simulink library "speedgoatlib_IO71X"  (R2012b)
settings: Solver=ode45  StartTime=0.0  StopTime=10.0  RelTol=1e-3
undefined symbols (not defined in the file): macaddr
Description:
  | 7.14.0.739 (R2012a)
settings Model: xpc_rtwmakecfg_data=_xpciplib__xpcetherlib__xpcether8255xlib__xpcnblib__xpcetherGbElib_  Creator=dkuratli  LastModifiedBy=lab3

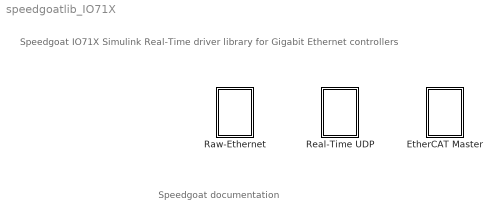
== system speedgoatlib_IO71X ==
  note: Speedgoat IO71X Simulink Real-Time driver library
      | for Gigabit Ethernet controllers
  note: Speedgoat documentation
  EtherCAT Master : Subsystem
      settings: OpenFcn=xpcethercatlib
  Raw-Ethernet : Subsystem
      settings: OpenFcn=xpcethernetlib
  Real-Time UDP : Subsystem

== system speedgoatlib_IO71X/EtherCAT Master ==

== system speedgoatlib_IO71X/Raw-Ethernet ==

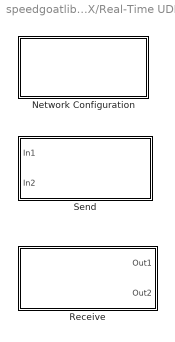
== system speedgoatlib_IO71X/Real-Time UDP ==
  "Network Configuration " : Subsystem  mask(xpcnwconfig){EthController=1, IpAddress=0.0.0.0, SubnetMask=255.255.255.0, Gateway=0.0.0.0, EthDrv=Intel Gigabit, PciBus=0, PciSlot=0, BufferSizes=[100 10 10 200]}
      mask prompts: EthController "Ethernet controller"; IpAddress "IP Address:"; SubnetMask "Subnet Mask:"; EthDrv "Ethernet Driver"; PciBus "PCI Bus:"; PciSlot "PCI Slot:"; BufferSizes "Buffer pool sizes (256, 512, 1024, 2048)"
      mask help: Network Configuration
      mask init:
      | EthDrv = 2;
      | IpAddress = ipaddr(IpAddress);
      | SubnetMask = ipaddr(SubnetMask);
      | Gateway = ipaddr(Gateway);
      mask Help: eval('xpcdoc(''RT_NETWORK_CONFIGURATION'')');
      mask TypeOptions EthController: 1 | 2 | 3 | 4 | 5 | 6 | 7 | 8 | 9 | 10
      mask TypeOptions EthDrv: Intel 8255x | Intel Gigabit
      mask Display: disp(['Speedgoat\nI8254x (IO71X)\nNetwork Configuration\nEthernet controller: ', num2str(EthController)]);
  "Receive " : Subsystem  mask(receive){EthController=1, Receive1=0.0.0.0, Receive2=25000, Receive3=1, Receive4=-1}
      mask prompts: EthController "Ethernet controller:"; Receive1 "IP address to receive from (0.0.0.0 for accepting all):"; Receive2 "IP port to receive from:"; Receive3 "Output port width:"; Receive4 "Sample time:"
      mask help: UDP Receive (adapted by Speedgoat)
      mask init:
      | Receive1 = ipaddr(Receive1);
      mask Help: helpview(fullfile(docroot, 'mapfiles', 'xpc.map'), 'RT_UDP_RECEIVE')
      mask TypeOptions EthController: 1 | 2 | 3 | 4 | 5 | 6 | 7 | 8 | 9 | 10
      mask Display: disp(['Speedgoat\nI8254x (IO71X)\nUDP Receive\nEthernet controller: ', num2str(EthController)])
  "Send " : Subsystem  mask(send){EthController=1, Send1=255.255.255.255, Send2=25000, Send3=-1, Send4=-1}
      mask prompts: EthController "Ethernet controller:"; Send1 "IP address to send to (255.255.255.255 for broadcast):"; Send2 "Remote IP port to send to:"; Send3 "Use the following local IP port (-1 for automatic assignment):"; Send4 "Sample time:"
      mask help: UDP Send (adapted by Speedgoat)
      mask init:
      | Send1 = ipaddr(Send1);
      mask Help: helpview(fullfile(docroot, 'mapfiles', 'xpc.map'), 'RT_UDP_SEND')
      mask TypeOptions EthController: 1 | 2 | 3 | 4 | 5 | 6 | 7 | 8 | 9 | 10
      mask Display: disp(['Speedgoat\nI8254x (IO71X)\nUDP Send\nEthernet controller: ',num2str(EthController)])

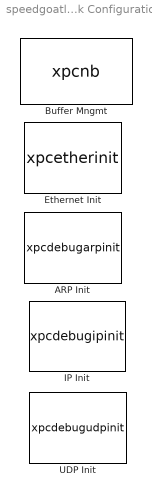
== system speedgoatlib_IO71X/Real-Time UDP/Network Configuration  ==
  "ARP Init " : S-Function  Priority=0  FunctionName=xpcdebugarpinit  Parameters=Stats, Interface, IpAddress, SubnetMask, Gateway, EthernetId, Flags, BlockId, Retry, Timeout, Expiration, StaticAddressListIp, StaticAddressListMac, DiscoveryList, MulticastList, SampleTime  EnableBusSupport=off  mask(arpinit){Interface=EthController-1, IpAddress=IpAddress, SubnetMask=SubnetMask, Gateway=Gateway, EthernetId=EthController, BlockId=EthController-1, SampleTime=-1, Flags=hex2dec('00000697'), Stats=off, Retry=5, Timeout=20, Expiration=20*60, StaticAddressListIp=[], StaticAddressListMac=[], DiscoveryList=[], MulticastList=[]}
      mask prompts: IpAddress "IP Address"; SubnetMask "Subnet Mask"; EthernetId "Ethernet ID"; BlockId "Block ID"; SampleTime "Sample Time"; Stats "Statistics Port"; StaticAddressListIp "[Static IP]"; StaticAddressListMac "[Static MAC]"; DiscoveryList "[Discovery IP]"; MulticastList "[Multicast IP]"
      mask help: ARP Init
      mask init:
      | xpclinklib('xpciplib');
      mask Help: web('arpdebug.htm',  '-helpbrowser');
      mask Display: disp('ARP Init');
  "Buffer Mngmt " : S-Function  Priority=-1  FunctionName=xpcnb  Parameters=pool_sizes, SampleTime, ShowTune  EnableBusSupport=off  mask(xpcnbinit){SampleTime=-1, PoolSizes=BufferSizes, ShowTune=on}
      mask prompts: SampleTime "Sample time:"; PoolSizes "Buffer pool sizes (256, 512, 1024, 2048):"; ShowTune "Display tuning information"
      mask help: Network Buffer Initialization
      mask init:
      | [MaskDisplay, pool_sizes] = mxpcnbinit(2, PoolSizes);
      | 
      | set_param(gcb, 'MaskDisplay', MaskDisplay);
      mask Help: eval('xpcdoc(''NB_Init'')');
      mask Display: disp('Network Buffer\nManagement');
  "Ethernet Init " : S-Function  Priority=-1  FunctionName=xpcetherinit  Parameters="ID, Driver, Bus, Slot, VendorID, DeviceID, AddressSource, mac, TxSA, RxPromiscuous, RxBad, RxShort, MaxMTU, TxThreshold, TxBuffers, RxBuffers, ShowTune, numMulti, multicast,   NumRxBlks, SampleTime"  EnableBusSupport=off  mask(xpcetherinit){ID=EthController, Driver=EthDrv, Bus=PciBus, Slot=PciSlot, SampleTime=-1, AddressSource=EEPROM, MAC=macaddr('00:00:00:00:00:00'), TxSA=off, RxPromiscuous=off, Multicast={}, RxBad=off, RxShort=off, MaxMTU=1518, TxThreshold=224, TxBuffers=128, RxBuffers=64, ShowTune=off, NumRxBlks=1}
      mask prompts: ID "Device ID:"; Bus "PCI bus:"; Slot "PCI slot:"; SampleTime "Sample time:"; AddressSource "Address source:"; TxSA "Tx source address from model"; RxPromiscuous "Rx promiscuous"; Multicast "Multicast address list:"; RxBad "Rx bad frames"; RxShort "Rx short frames"; MaxMTU "Max MTU:"; TxThreshold "Tx threshold:"; TxBuffers "Tx buffers:"; RxBuffers "Rx buffers:"; ShowTune "Display tuning information"; NumRxBlks "num rx blocks"
      mask help: Ethernet Initialization
      mask init:
      | VendorID = -1;
      | DeviceID = -1;
      | 
      | [MaskDisplay, VendorID, DeviceID, mac, numMulti, multicast] = mxpcetherinit(2, ID, Driver, Bus, Slot, MAC, Multicast);
      | 
      | set_param(gcb, 'MaskDisplay', MaskDisplay);
      mask Help: eval('xpcdoc(''Ether_Init'')');
      mask TypeOptions AddressSource: EEPROM | Specify
      mask Callback AddressSource:
      | enables = get_param(gcb, 'MaskVisibilities');
      | if strcmp('Specify', get_param(gcb, 'AddressSource'))
      |     enables{strmatch('MAC',fieldnames(get_param(gcb,'DialogParameters')))} = 'on';
      | else
      |     enables{strmatch('MAC',fieldnames(get_param(gcb,'DialogParameters')))} = 'off';
      | end
      | set_param(gcb, 'MaskVisibilities', enables);
      mask Display: disp('Ethernet\nInitialization\nbus: 0 slot: 0\nId: 1\n');
  "IP Init " : S-Function  Priority=1  FunctionName=xpcdebugipinit  Parameters=Stats, Group, ArpId, IpAddress, SubnetMask, DefaultGateway, DefaultInterface, Flags, ToS, StartingId, TTL, SampleTime  EnableBusSupport=off  mask(ipinit){Group=EthController-1, ArpId=EthController-1, IpAddress=[IpAddress], SubnetMask=[SubnetMask], DefaultGateway=Gateway, DefaultInterface=0, SampleTime=-1, Flags=hex2dec('00000005'), ToS=hex2dec('00'), StartingId=10000, TTL=64, Stats=off}
      mask prompts: ArpId "[ARP ID]"; IpAddress "[IP Address]"; SubnetMask "[Subnet Mask]"; DefaultGateway "Default Gateway"; DefaultInterface "Default Interface"; SampleTime "Sample Time"; StartingId "Starting Id"; Stats "Statistics Port"
      mask help: IP Init
      mask init:
      | xpclinklib('xpciplib');
      mask Help: web('ipdebug.htm',  '-helpbrowser');
      mask Display: disp('IP Init');
  "UDP Init " : S-Function  Priority=2  FunctionName=xpcdebugudpinit  Parameters=Stats, Group, StartingPort, Flags, SampleTime  EnableBusSupport=off  mask(udpinit){Group=EthController-1, StartingPort=10000, Flags=hex2dec('00000001'), SampleTime=-1, Stats=off}
      mask prompts: StartingPort "Starting Port"; SampleTime "Sample Time"; Stats "Statistics Port"
      mask help: UDP Init
      mask init:
      | xpclinklib('xpciplib');
      mask Help: web('udpdebug.htm',  '-helpbrowser');
      mask Display: disp('UDP Init');

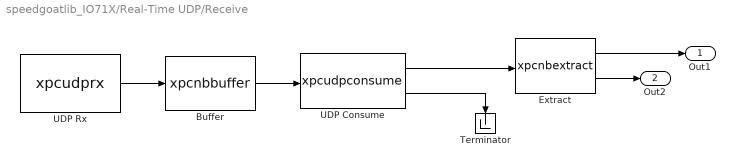
== system speedgoatlib_IO71X/Real-Time UDP/Receive  ==
  "Buffer " : S-Function  FunctionName=xpcnbbuffer  Parameters=chainSize, bufferSize, Threshold  EnableBusSupport=off  mask(xpcnbbuffer){ChainSize=1, BufferSize=2, Threshold=0}
      mask prompts: ChainSize "Chain size:"; BufferSize "Buffer size:"
      mask help:
      | Network Buffer Buffering
      |
      | Chain size = inf --> No buffering, all packets passed through
      | Chain size = 0   --> Deletes all packets, none passed through
      | Chain size > 0   --> Passes through first "Chain size" packets
      | Chain size < 0   --> Passes through last "Chain size" packets
      |
      | Buffer size = inf --> All remaining packets are buffered, none are deleted
      | Buffer size = 0   --> No buffering, deletes all remaining packets
      | Buffer size > 0   --> Buffers remaining first "Buffer size" packets
      | Buffer size < 0   --> Buffers remaining last "Buffer size" packets
      |
      | Threshold = 0 --> No threshold
      | Threshold > 0 --> Delay passing through packets till threshold is met once
      | Threshold < 0 --> Passes through packets if "Threshold" packets are buffered
      mask init:
      | [MaskDisplay, chainSize, bufferSize] = mxpcnbbuffer(2, ChainSize, BufferSize, Threshold);
      | 
      | set_param(gcb, 'MaskDisplay', MaskDisplay);
      mask Help: helpview(fullfile(docroot, 'mapfiles', 'xpc.map'), 'NB_Buffer')
      mask Display: disp('NB\nBuffering\n\n2');port_label('output', 1, '1');
  "Extract " : S-Function  FunctionName=xpcnbextract  Parameters=packetSize  EnableBusSupport=off  mask(xpcnbextract){PacketSize=Receive3}
      mask prompts: PacketSize "Packet size (-1: inherit):"
      mask help: Network Buffer Extract
      mask init:
      | [packetSize] = mxpcnbextract(2,PacketSize);
      mask Help: helpview(fullfile(docroot, 'mapfiles', 'xpc.map'), 'NB_Extract')
      mask Display: disp('NB Extract\n');port_label('output', 2, 'length');
  Terminator : Terminator
  "UDP Consume " : S-Function  FunctionName=xpcudpconsume  Parameters=Group, VectorSize, SampleTime  EnableBusSupport=off  mask(udpconsume){Group=0, VectorSize=0, SampleTime=Receive4}
      mask prompts: Group "IP Group"; VectorSize "Output port width:"; SampleTime "Sample time:"
      mask help: UDP Consume
      mask Help: helpview(fullfile(docroot, 'mapfiles', 'xpc.map'), 'RT_UDP_CONSUME')
      mask Display:
      | if VectorSize
      |     disp('UDP Consume\n\n\n\n\n\n\n');
      |     port_label('output', 1, 'Buffers');
      |     port_label('output', 2, 'Source IP Address');
      |     port_label('output', 3, 'Destination IP Address');
      |     port_label('output', 4, 'Local UDP Port');
      |     port_label('output', 5, 'Remote UDP Port');
      |     port_label('output', 6, 'Chain Size');
      | else
      |     disp('UDP Consume');
      |     port_label('output', 1, 'Buffers');
      |     port_label('output', 2, 'Chain Size');
      | end
  "UDP Rx " : S-Function  Priority=5  FunctionName=xpcudprx  Parameters=Group, SourceAddress, sip, LocalPort, lup, SampleTime  EnableBusSupport=off  mask(udprx){Group=EthController-1, sip=Any, SourceAddress=Receive1, lup=Specify, LocalPort=Receive2, SampleTime=Receive4}
      mask prompts: Group "IP Group"; sip "Source IP Address"; SourceAddress "IP address to receive from (0.0.0.0 for accepting all):"; lup "Local UDP Port"; LocalPort "IP port to receive from:"; SampleTime "Sample time:"
      mask help: UDP Rx
      mask init:
      | if SourceAddress == 0
      |     sip = 3;
      | else
      |     sip = 1;
      | end
      mask Help: helpview(fullfile(docroot, 'mapfiles', 'xpc.map'), 'RT_UDP_RX')
      mask TypeOptions sip: Specify | Port | Any
      mask TypeOptions lup: Specify | Port | Any
      mask Display: disp('UDP Rx');
  Out1 : Outport  OutDataTypeStr=uint8
  Out2 : Outport  Port=2  OutDataTypeStr=double
  wires:
  "UDP Consume "/2 -> Terminator/1
  "UDP Consume "/1 -> "Extract "/1
  "UDP Rx "/1 -> "Buffer "/1
  "Buffer "/1 -> "UDP Consume "/1
  "Extract "/1 -> Out1/1
  "Extract "/2 -> Out2/1

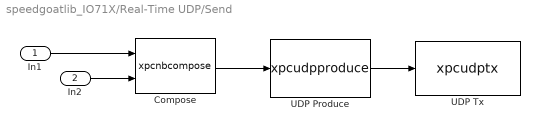
== system speedgoatlib_IO71X/Real-Time UDP/Send  ==
  In1 : Inport  OutDataTypeStr=uint8
  In2 : Inport  Port=2  OutDataTypeStr=double
  "Compose " : S-Function  FunctionName=xpcnbcompose  EnableBusSupport=off  mask(xpcnbcompose){}
      mask help: Network Buffer Compose
      mask init:
      | mxpcnbcompose(2);
      mask Help: helpview(fullfile(docroot, 'mapfiles', 'xpc.map'), 'NB_Compose')
      mask Display: disp('NB Compose\n');port_label('input', 2, 'length');
  "UDP Produce " : S-Function  Priority=5  FunctionName=xpcudpproduce  Parameters=Group, SrcIp, sip, DstIp, dip, LocPort, lup, RemPort, rup, SampleTime  EnableBusSupport=off  mask(udpproduce){Group=EthController-1, sip=Auto, SrcIp=0.0.0.0, dip=Specify, DstIp=Send1, rup=Specify, RemPort=Send2, lup=Auto, LocPort=Send3, SampleTime=Send4}
      mask prompts: Group "IP Group"; sip "Source IP Address"; SrcIp "Source IP Address"; dip "Destination IP Address"; DstIp "IP address to send to (255.255.255.255 for broadcast):"; rup "Remote UDP Port"; RemPort "Remote IP port to send to:"; lup "Local UDP Port"; LocPort "Use the following local IP port (-1 for automatic assignment):"; SampleTime "Sample time:"
      mask help: UDP Produce
      mask init:
      | if LocPort == -1
      |     lup = 3;
      | else
      |     lup = 1;
      | end
      | 
      | SrcIp = ipaddr(SrcIp);
      | DstIp = ipaddr(DstIp);
      mask Help: helpview(fullfile(docroot, 'mapfiles', 'xpc.map'), 'RT_UDP_PRODUCE')
      mask TypeOptions sip: Specify | Port | Auto
      mask TypeOptions dip: Specify | Port
      mask TypeOptions rup: Specify | Port
      mask TypeOptions lup: Specify | Port | Auto
      mask Display: disp('UDP Produce');
  "UDP Tx " : S-Function  Priority=5  FunctionName=xpcudptx  Parameters=Group, TTL, ToS, SampleTime  EnableBusSupport=off  mask(udptx){Group=EthController-1, TTL=-1, ToS=-1, SampleTime=Send4}
      mask prompts: Group "IP Group"; SampleTime "Sample Time"
      mask help: UDP Tx
      mask Help: eval('xpcdoc(''RT_UDP_TX'')');
      mask Display: disp('UDP Tx');
  wires:
  "UDP Produce "/1 -> "UDP Tx "/1
  "Compose "/1 -> "UDP Produce "/1
  In1/1 -> "Compose "/1
  In2/1 -> "Compose "/2
